simulink model "BLDC_simulink"  (R2015b)
settings: Solver=VariableStepAuto  StartTime=0.0  StopTime=50  RelTol=1e-3
values from neighbouring files (symbols this model uses):
  A_motor = [-137362.637363 0 0 0 0 -137362.637363 0 0 0 0 -3.96e-07 1 ... (16 elements, 4x4)]    [BLDC.mat]    (also in bldc_maybe.mat = [-416.666666667 0 0 0 0 -416.666666667 0 0 0 0 0 1 ... (16 e)
  B_motor = [7326.00732601  3663.003663  0; -3663.003663  3663.003663  0; 0  0  20; 0  0  0]    [BLDC.mat]    (also in bldc_maybe.mat)
  C_motor = [1 0 0 0 0 1 0 0 0 0 1 0 ... (16 elements, 4x4)]    [BLDC.mat]    (also in bldc_maybe.mat)
  D_motor = [0  0  0; 0  0  0; 0  0  0; 0  0  0]    [BLDC.mat]    (also in bldc_maybe.mat)
  Ke = 1.05    [BLDC.mat]    (also in bldc_maybe.mat)
  Kt = 1.05    [BLDC.mat]    (also in bldc_maybe.mat)
libraries: powerlib x14, simulink x1
settings Model: Creator=Jana  LastModifiedBy=Jana

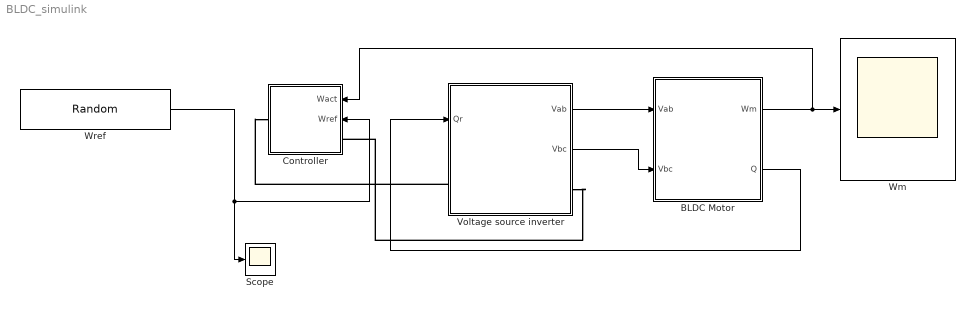
== system BLDC_simulink ==
  BLDC Motor : Subsystem
  Controller : Subsystem
  Scope : Scope
  Voltage source inverter : Subsystem
  Wm : Scope
  Wref : RandomNumber  Mean=10  Variance=60  SampleTime=6
  wires:
  BLDC Motor/1(Wm) -> Controller/1(Wact), Wm/1
  Voltage source inverter/1(Vab) -> BLDC Motor/1(Vab)
  Voltage source inverter/2(Vbc) -> BLDC Motor/2(Vbc)
  BLDC Motor/2(Q) -> Voltage source inverter/1(Qr)
  Wref/1 -> Scope/1, Controller/2(Wref)
  connections:
  Voltage source inverter/LConn1 -- Controller/RConn1
  Voltage source inverter/RConn1 -- Controller/LConn1

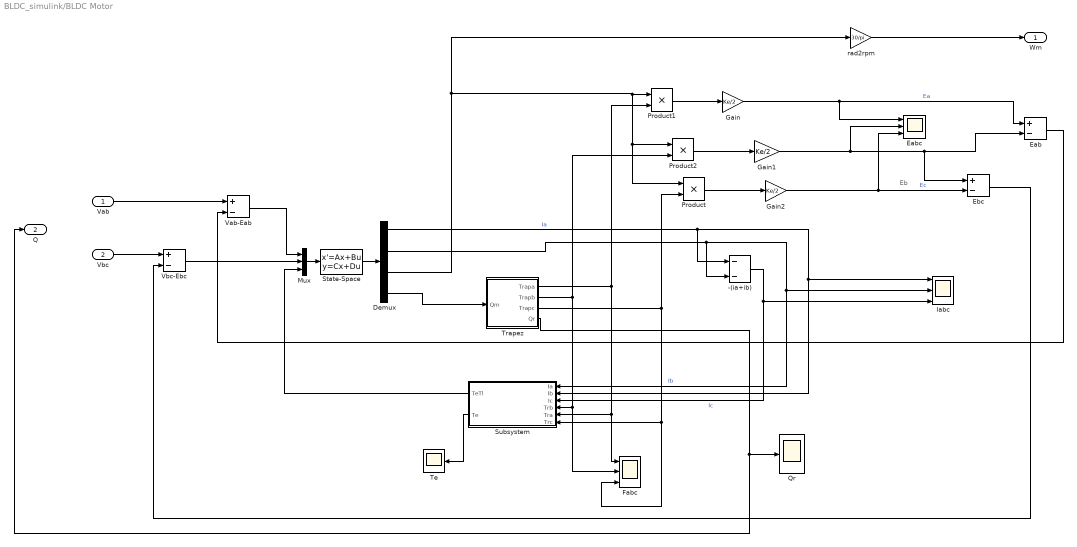
== system BLDC_simulink/BLDC Motor ==
  note: Eb
  Vab : Inport
  Vbc : Inport  Port=2
  -(ia+ib) : Sum  Inputs=--
  Demux : Demux
  Eab : Sum  Inputs=+-
  Eabc : Scope  NumInputPorts=3
  Ebc : Sum  Inputs=+-
  Fabc : Scope  NumInputPorts=3
  Gain : Gain  Gain=Ke/2
  Gain1 : Gain  Gain=Ke/2
  Gain2 : Gain  Gain=Ke/2
  Iabc : Scope  NumInputPorts=3
  Mux : Mux  Inputs=3
  Product : Product
  Product1 : Product
  Product2 : Product
  Qr : Scope
  State-Space : StateSpace  A=A_motor  B=B_motor  C=C_motor  D=D_motor  X0=0  ContinuousStateAttributes='Angularspeed'
  Subsystem : Subsystem
  Te : Scope
  Trapez : Subsystem
  Vab-Eab : Sum  Inputs=+-
  Vbc-Ebc : Sum  Inputs=+-
  rad2rpm : Gain  Gain=30/pi
  Wm : Outport
  Q : Outport  Port=2
  wires:
  Ebc/1 -> Vbc-Ebc/2
  Vab-Eab/1 -> Mux/1
  Vbc-Ebc/1 -> Mux/2
  Eab/1 -> Vab-Eab/2
  Demux/4 -> Trapez/1(Qm)
  Gain1/1 -> Eab/2, Ebc/1, Eabc/2
  Demux/3 -> Product2/1, Product/1, Product1/1, rad2rpm/1
  Subsystem/2(Te) -> Te/1
  Mux/1 -> State-Space/1
  Demux/2 -> Subsystem/1(Ia), Iabc/2, -(ia+ib)/2  "Ib"
  -(ia+ib)/1 -> Subsystem/3(Ic), Iabc/3  "Ic"
  Trapez/1(Trapa) -> Product1/2, Fabc/1, Subsystem/5(Tra)
  Product2/1 -> Gain1/1
  Demux/1 -> Iabc/1, Subsystem/2(Ib), -(ia+ib)/1  "Ia"
  Trapez/3(Trapc) -> Fabc/3, Subsystem/6(Trc), Product/2
  Product/1 -> Gain2/1
  Trapez/2(Trapb) -> Fabc/2, Subsystem/4(Trb), Product2/2
  Subsystem/1(TeTl) -> Mux/3
  Gain/1 -> Eab/1, Eabc/1  "Ea"
  State-Space/1 -> Demux/1
  Trapez/4(Qr) -> Qr/1, Q/1
  Product1/1 -> Gain/1
  Gain2/1 -> Ebc/2, Eabc/3  "Ec"
  rad2rpm/1 -> Wm/1
  Vbc/1 -> Vbc-Ebc/1
  Vab/1 -> Vab-Eab/1

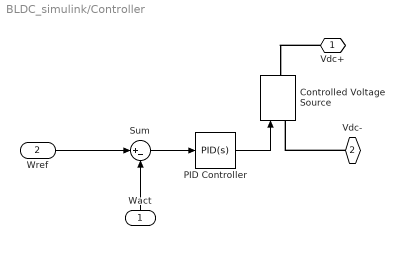
== system BLDC_simulink/Controller ==
  Wact : Inport
  Wref : Inport  Port=2
  Controlled Voltage Source : powerlib/Electrical Sources/Controlled Voltage Source  Initialize=on  Source_Type=AC  Amplitude=0  Phase=0  Frequency=0  Measurements=None
  PID Controller : simulink/Continuous/PID Controller  Controller=PID  TimeDomain=Continuous-time  SampleTime=-1  IntegratorMethod=Forward Euler  FilterMethod=Forward Euler  Form=Parallel  UseFilter=on  ControllerParametersSource=internal  P=9  I=0.015  D=0.6  N=100  InitialConditionSource=internal  InitialConditionForIntegrator=0  InitialConditionForFilter=0  ExternalReset=none  LimitOutput=off  UpperSaturationLimit=inf  LowerSaturationLimit=-inf  LinearizeAsGain=on  AntiWindupMode=none  Kb=1  TrackingMode=off  Kt=1  PParamMin=[]  PParamMax=[]  IParamMin=[]  IParamMax=[]  DParamMin=[]  DParamMax=[]  NParamMin=[]  NParamMax=[]  KbParamMin=[]  KbParamMax=[]  KtParamMin=[]  KtParamMax=[]  POutMin=[]  POutMax=[]  IOutMin=[]  IOutMax=[]  DOutMin=[]  DOutMax=[]  NOutMin=[]  NOutMax=[]  KbOutMin=[]  KbOutMax=[]  KtOutMin=[]  KtOutMax=[]  IntegratorOutMin=[]  IntegratorOutMax=[]  FilterOutMin=[]  FilterOutMax=[]  SumOutMin=[]  SumOutMax=[]  SumI1OutMin=[]  SumI1OutMax=[]  SumI2OutMin=[]  SumI2OutMax=[]  SumI3OutMin=[]  SumI3OutMax=[]  SumDOutMin=[]  SumDOutMax=[]  SaturationOutMin=[]  SaturationOutMax=[]  IntegratorContinuousStateAttributes=''  IntegratorStateMustResolveToSignalObject=off  IntegratorRTWStateStorageClass=Auto  FilterContinuousStateAttributes=''  FilterStateMustResolveToSignalObject=off  FilterRTWStateStorageClass=Auto  DifferentiatorICPrevScaledInput=0  DifferentiatorOutMin=[]  DifferentiatorOutMax=[]
  Sum : Sum  Inputs=|+-
  Vdc+ : PMIOPort  Port=1  Side=Right
  Vdc- : PMIOPort  Port=2  Side=Left
  wires:
  Wact/1 -> Sum/2
  PID Controller/1 -> Controlled Voltage Source/1
  Sum/1 -> PID Controller/1
  Wref/1 -> Sum/1
  connections:
  Vdc+/RConn1 -- Controlled Voltage Source/RConn1
  Vdc-/RConn1 -- Controlled Voltage Source/LConn1

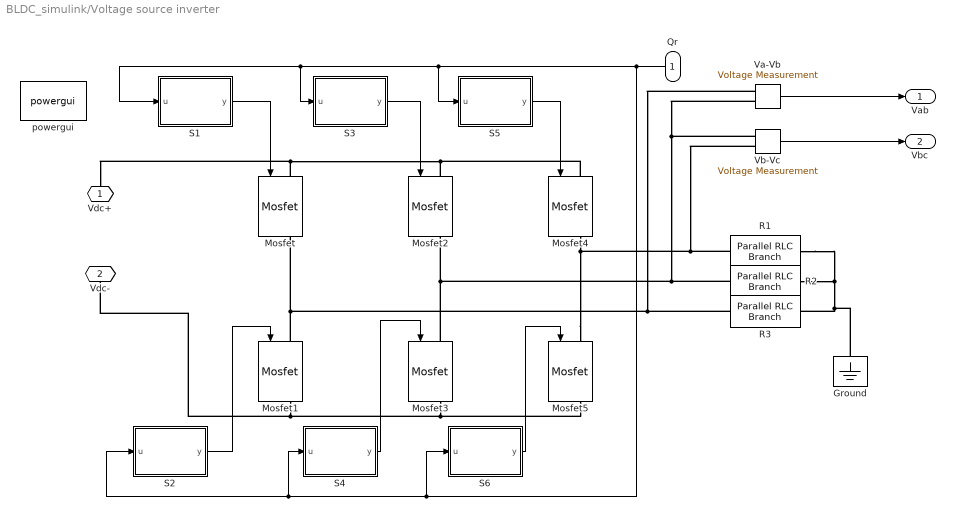
== system BLDC_simulink/Voltage source inverter ==
  Qr : Inport
  Ground : powerlib/Elements/Ground  LConnTagsString=a
  Mosfet{,1..5} (6 alike) : powerlib/Power Electronics/Mosfet  Ron=0.1  Lon=0  Rd=0.01  Vfd=0  IC=0  Rs=1e5  Cs=inf  Measurements=on
  R1 : powerlib/Elements/Parallel RLC Branch  LConnTagsString=a  RConnTagsString=__new0  BranchType=R  Resistance=1  Inductance=1e-3  SetiL0=off  InitialCurrent=0  Capacitance=1e-6  Setx0=off  InitialVoltage=0  Measurements=None
  R2 : powerlib/Elements/Parallel RLC Branch  LConnTagsString=a  RConnTagsString=__new0  BranchType=R  Resistance=1  Inductance=1e-3  SetiL0=off  InitialCurrent=0  Capacitance=1e-6  Setx0=off  InitialVoltage=0  Measurements=None
  R3 : powerlib/Elements/Parallel RLC Branch  LConnTagsString=a  RConnTagsString=__new0  BranchType=R  Resistance=1  Inductance=1e-3  SetiL0=off  InitialCurrent=0  Capacitance=1e-6  Setx0=off  InitialVoltage=0  Measurements=None
  S1 : MATLAB Function  TreatAsAtomicUnit=on
  S2 : MATLAB Function  TreatAsAtomicUnit=on
  S3 : MATLAB Function  TreatAsAtomicUnit=on
  S4 : MATLAB Function  TreatAsAtomicUnit=on
  S5 : MATLAB Function  TreatAsAtomicUnit=on
  S6 : MATLAB Function  TreatAsAtomicUnit=on
  Va-Vb : powerlib/Measurements/Voltage Measurement  PhasorSimulation=off  OutputType=Complex  PSBequivalent=0
  Vb-Vc : powerlib/Measurements/Voltage Measurement  PhasorSimulation=off  OutputType=Complex  PSBequivalent=0
  powergui : powerlib/powergui  Priority=1  SimulationMode=Continuous  SolverType=Tustin/Backward Euler (TBE)  SampleTime=50e-6  frequency=60  SPID=off  DisableSnubberDevices=off  DisableRonSwitches=off  DisableVfSwitches=off  SwTol=0  DisplayEquations=off  Interpol=off  ExternalGateDelay=off  methode=off  Ts=10  FunctionMessages=off  echomessages=off  HookPort=off  EnableUseOfTLC=off  x0status=blocks  frequencyindice=0  Pbase=100e6  ErrMax=1e-4  Iterations=50  UnitsV=kV  UnitsW=MW  buscounter=0  RestoreLinks=warning  ResistiveCurrentMeasurement=off  Frange=[0:2:500]  Ylog=off  Xlog=on  ShowGrid=off  save=off  variable=ZData  structure=0  ZoomFFT=off  StartTime=0.0  cycles=1  DisplayStyle=1  fundamental=60  FreqAxis=off  MaxFrequency=1000  frequencyindicesteady=1  RmsSteady=1  display=off
  Vdc+ : PMIOPort  Port=1  Side=Left
  Vdc- : PMIOPort  Port=2  Side=Right
  Vab : Outport
  Vbc : Outport  Port=2
  wires:
  S5/1(y) -> Mosfet4/1
  S3/1(y) -> Mosfet2/1
  S2/1(y) -> Mosfet1/1
  Va-Vb/1 -> Vab/1
  S4/1(y) -> Mosfet3/1
  S6/1(y) -> Mosfet5/1
  S1/1(y) -> Mosfet/1
  Vb-Vc/1 -> Vbc/1
  Qr/1 -> S3/1(u), S1/1(u), S5/1(u), S2/1(u), S4/1(u), S6/1(u)
  connections:
  Mosfet5/LConn1 -- Vb-Vc/LConn2 -- R1/LConn1 -- Mosfet4/RConn1
  Mosfet2/LConn1 -- Vdc+/RConn1 -- Mosfet/LConn1 -- Mosfet4/LConn1
  Mosfet3/RConn1 -- Mosfet5/RConn1 -- Vdc-/RConn1 -- Mosfet1/RConn1
  Mosfet1/LConn1 -- Va-Vb/LConn1 -- R3/LConn1 -- Mosfet/RConn1
  R3/RConn1 -- R2/RConn1 -- R1/RConn1 -- Ground/LConn1
  Mosfet3/LConn1 -- Vb-Vc/LConn1 -- Va-Vb/LConn2 -- R2/LConn1 -- Mosfet2/RConn1

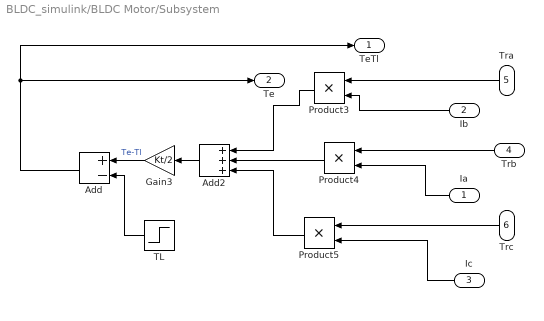
== system BLDC_simulink/BLDC Motor/Subsystem ==
  Ia : Inport
  Ib : Inport  Port=2
  Ic : Inport  Port=3
  Trb : Inport  Port=4
  Tra : Inport  Port=5
  Trc : Inport  Port=6
  Add : Sum  Inputs=+-
  Add2 : Sum  Inputs=+++
  Gain3 : Gain  Gain=Kt/2
  Product3 : Product
  Product4 : Product
  Product5 : Product
  TL : Step  After=0.2  SampleTime=0
  TeTl : Outport
  Te : Outport  Port=2
  wires:
  Trc/1 -> Product5/1
  Trb/1 -> Product4/1
  Ic/1 -> Product5/2
  Ib/1 -> Product3/2
  Tra/1 -> Product3/1
  Ia/1 -> Product4/2
  TL/1 -> Add/2
  Product4/1 -> Add2/2
  Product5/1 -> Add2/3
  Add2/1 -> Gain3/1
  Product3/1 -> Add2/1
  Gain3/1 -> Add/1  "Te-Tl"
  Add/1 -> TeTl/1, Te/1

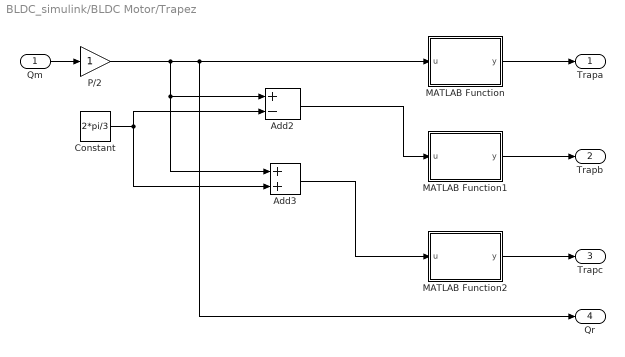
== system BLDC_simulink/BLDC Motor/Trapez ==
  Qm : Inport
  Add2 : Sum  Inputs=+-
  Add3 : Sum
  Constant : Constant  Value=2*pi/3
  MATLAB Function : MATLAB Function  TreatAsAtomicUnit=on
  MATLAB Function1 : MATLAB Function  TreatAsAtomicUnit=on
  MATLAB Function2 : MATLAB Function  TreatAsAtomicUnit=on
  P/2 : Gain
  Trapa : Outport
  Trapb : Outport  Port=2
  Trapc : Outport  Port=3
  Qr : Outport  Port=4
  wires:
  MATLAB Function1/1(y) -> Trapb/1
  Qm/1 -> P/2/1
  Add2/1 -> MATLAB Function1/1(u)
  MATLAB Function2/1(y) -> Trapc/1
  MATLAB Function/1(y) -> Trapa/1
  Constant/1 -> Add2/2, Add3/2
  P/2/1 -> MATLAB Function/1(u), Qr/1, Add3/1, Add2/1
  Add3/1 -> MATLAB Function2/1(u)

== matlab function BLDC_simulink/BLDC Motor/Trapez/MATLAB Function1 ==
  data: u input; y output
function y = fcn(u)
%#codegen
Q = mod(u,2*pi);
if Q<2*pi/3    
    T = 1;
elseif Q < pi
    T = 1-6*(Q-2*pi/3)/pi;
elseif Q < 5*pi/3
    T = -1;
elseif Q < 2*pi
    T = -1 + 6*(Q-5*pi/3)/pi;
else
    T = nan;   %if data was inf or nan
end
y=T;

== matlab function BLDC_simulink/BLDC Motor/Trapez/MATLAB Function2 ==
  data: u input; y output
function y = fcn(u)
%#codegen
Q = mod(u,2*pi);
if Q<2*pi/3    
    T = 1;
elseif Q < pi
    T = 1-6*(Q-2*pi/3)/pi;
elseif Q < 5*pi/3
    T = -1;
elseif Q < 2*pi
    T = -1 + 6*(Q-5*pi/3)/pi;
else
    T = nan;   %if data was inf or nan
end
y=T;

== matlab function BLDC_simulink/Voltage source inverter/S1 ==
  data: u input; y output
function y = fcn(u)
%#codegen
u = rem(u,2*pi);
y =0;
if u >= 0 && u < 2*pi/3
    y =1;
end

== matlab function BLDC_simulink/BLDC Motor/Trapez/MATLAB Function ==
  data: u input; y output
function y = fcn(u)
%#codegen
Q = mod(u,2*pi);
if Q<2*pi/3    
    T = 1;
elseif Q < pi
    T = 1-6*(Q-2*pi/3)/pi;
elseif Q < 5*pi/3
    T = -1;
elseif Q < 2*pi
    T = -1 + 6*(Q-5*pi/3)/pi;
else
    T = nan;   %if data was inf or nan
end
y=T;

== matlab function BLDC_simulink/Voltage source inverter/S2 ==
  data: u input; y output
function y = fcn(u)
%#codegen
u = rem(u,2*pi);
y =0;
if u >= pi && u < 5*pi/3
    y =1;
end

== matlab function BLDC_simulink/Voltage source inverter/S3 ==
  data: u input; y output
function y = fcn(u)
%#codegen
u = rem(u,2*pi);
y =0;
if u >= 2*pi/3 && u < 4*pi/3
    y =1;
end

== matlab function BLDC_simulink/Voltage source inverter/S4 ==
  data: u input; y output
function y = fcn(u)
%#codegen
u = rem(u,2*pi);
y =0;
if u >= 0 && u < pi/3
    y =1;
elseif u >= 5*pi/3 && u < 2*pi
    y=1;
end

== matlab function BLDC_simulink/Voltage source inverter/S5 ==
  data: u input; y output
function y = fcn(u)
%#codegen
u = rem(u,2*pi);
y =0;
if u >= 4*pi/3 && u < 2*pi
    y =1;
end

== matlab function BLDC_simulink/Voltage source inverter/S6 ==
  data: u input; y output
function y = fcn(u)
%#codegen
u = rem(u,2*pi);
y =0;
if u >= pi/3 && u < pi
    y =1;
end
